simulink model "Model_Evaluation"  (R2021b)
settings: Solver=VariableStepAuto  StartTime=0.0  StopTime=10.0  RelTol=1e-3
settings Model: Creator=travispaul  LastModifiedBy=travispaul

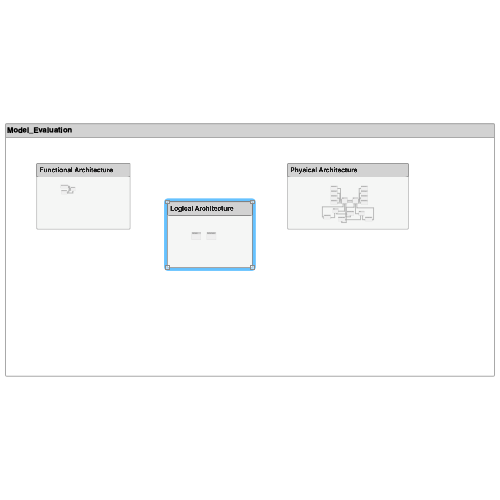
[thumbnail: Simulink's stored preview of the top-level diagram]
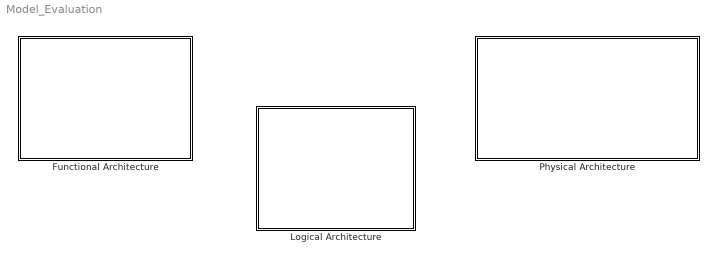
== system Model_Evaluation ==
  Functional Architecture : Subsystem
      settings: PortSchema="{\"entries\":[{\"content\":{\"headerSize\":26,\"margin\":15,\"minimumSpacing\":25,\"sides\":[{\"content\":{\"connectorIds\":[]},\"type\":\"ConnectorPlacement.EquallySpacedRectSide\",\"uuid\":\"40f43dd4-d871-4ec4-b3fe-13d7cd611bac\"},{\"content\":{\"connectorIds\":[],\"side\":\"RIGHT\"},\"type\":\"ConnectorPlacement.EquallySpacedRectSide\",\"uuid\":\"f931b331-3cfe-490c-8e42-e662817cbd7c\"},{\"content\":{\"connectorIds\":[],\"side\":\"TOP\"},\"type\":\"ConnectorPlacement.EquallySpacedRectSide\",\"uuid\":\"175320fb-a01d-4f5a-a2c2-6f21c6d50255\"}]},\"type\":\"ConnectorPlacement.EquallySpacedConnector\",\"uuid\":\"e178f2bb-de74-4782-8dfe-2993ee10560e\"}],\"packageUris\":[\"http://schema.mathworks.com/mf0/Connector/R2020b\"],\"version\":\"1.0\"}"
  Logical Architecture : Subsystem
      settings: PortSchema="{\"entries\":[{\"content\":{\"headerSize\":26,\"margin\":15,\"minimumSpacing\":25,\"sides\":[{\"content\":{\"connectorIds\":[]},\"type\":\"ConnectorPlacement.EquallySpacedRectSide\",\"uuid\":\"40f43dd4-d871-4ec4-b3fe-13d7cd611bac\"},{\"content\":{\"connectorIds\":[],\"side\":\"RIGHT\"},\"type\":\"ConnectorPlacement.EquallySpacedRectSide\",\"uuid\":\"f931b331-3cfe-490c-8e42-e662817cbd7c\"},{\"content\":{\"connectorIds\":[],\"side\":\"TOP\"},\"type\":\"ConnectorPlacement.EquallySpacedRectSide\",\"uuid\":\"175320fb-a01d-4f5a-a2c2-6f21c6d50255\"}]},\"type\":\"ConnectorPlacement.EquallySpacedConnector\",\"uuid\":\"e178f2bb-de74-4782-8dfe-2993ee10560e\"}],\"packageUris\":[\"http://schema.mathworks.com/mf0/Connector/R2020b\"],\"version\":\"1.0\"}"
  Physical Architecture : Subsystem
      settings: PortSchema="{\"entries\":[{\"content\":{\"headerSize\":26,\"margin\":15,\"minimumSpacing\":25,\"sides\":[{\"content\":{\"connectorIds\":[]},\"type\":\"ConnectorPlacement.EquallySpacedRectSide\",\"uuid\":\"40f43dd4-d871-4ec4-b3fe-13d7cd611bac\"},{\"content\":{\"connectorIds\":[],\"side\":\"RIGHT\"},\"type\":\"ConnectorPlacement.EquallySpacedRectSide\",\"uuid\":\"f931b331-3cfe-490c-8e42-e662817cbd7c\"},{\"content\":{\"connectorIds\":[],\"side\":\"TOP\"},\"type\":\"ConnectorPlacement.EquallySpacedRectSide\",\"uuid\":\"175320fb-a01d-4f5a-a2c2-6f21c6d50255\"}]},\"type\":\"ConnectorPlacement.EquallySpacedConnector\",\"uuid\":\"e178f2bb-de74-4782-8dfe-2993ee10560e\"}],\"packageUris\":[\"http://schema.mathworks.com/mf0/Connector/R2020b\"],\"version\":\"1.0\"}"

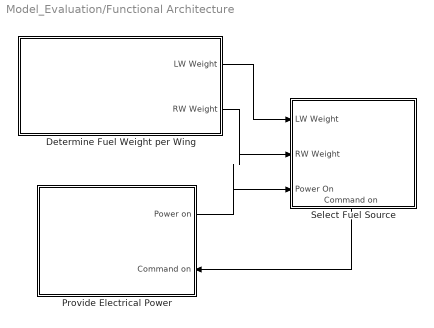
== system Model_Evaluation/Functional Architecture ==
  " Determine Fuel Weight per Wing" : Subsystem
      settings: PortSchema="{\"entries\":[{\"content\":{\"headerSize\":26,\"margin\":15,\"minimumSpacing\":25,\"sides\":[{\"content\":{\"connectorIds\":[]},\"type\":\"ConnectorPlacement.EquallySpacedRectSide\",\"uuid\":\"40f43dd4-d871-4ec4-b3fe-13d7cd611bac\"},{\"content\":{\"connectorIds\":[\"Out1\",\"Out2\"],\"side\":\"RIGHT\"},\"type\":\"ConnectorPlacement.EquallySpacedRectSide\",\"uuid\":\"f931b331-3cfe-490c-8e42-e662817cbd7c\"},{\"content\":{\"connectorIds\":[],\"side\":\"TOP\"},\"type\":\"ConnectorPlacement.EquallySpacedRectSide\",\"uuid\":\"175320fb-a01d-4f5a-a2c2-6f21c6d50255\"}]},\"type\":\"ConnectorPlacement.EquallySpacedConnector\",\"uuid\":\"e178f2bb-de74-4782-8dfe-2993ee10560e\"}],\"packageUris\":[\"http://schema.mathworks.com/mf0/Connector/R2020b\"],\"version\":\"1.0\"}"
  Provide Electrical Power : Subsystem
      settings: PortSchema="{\"entries\":[{\"content\":{\"headerSize\":26,\"margin\":15,\"minimumSpacing\":25,\"sides\":[{\"content\":{\"connectorIds\":[]},\"type\":\"ConnectorPlacement.EquallySpacedRectSide\",\"uuid\":\"40f43dd4-d871-4ec4-b3fe-13d7cd611bac\"},{\"content\":{\"connectorIds\":[\"Out1\",\"In1\"],\"side\":\"RIGHT\"},\"type\":\"ConnectorPlacement.EquallySpacedRectSide\",\"uuid\":\"f931b331-3cfe-490c-8e42-e662817cbd7c\"},{\"content\":{\"connectorIds\":[],\"side\":\"TOP\"},\"type\":\"ConnectorPlacement.EquallySpacedRectSide\",\"uuid\":\"175320fb-a01d-4f5a-a2c2-6f21c6d50255\"}]},\"type\":\"ConnectorPlacement.EquallySpacedConnector\",\"uuid\":\"e178f2bb-de74-4782-8dfe-2993ee10560e\"}],\"packageUris\":[\"http://schema.mathworks.com/mf0/Connector/R2020b\"],\"version\":\"1.0\"}"
  Select Fuel Source : Subsystem
      settings: PortSchema="{\"entries\":[{\"content\":{\"headerSize\":26,\"margin\":15,\"minimumSpacing\":25,\"sides\":[{\"content\":{\"connectorIds\":[\"In1\",\"In2\",\"In3\"]},\"type\":\"ConnectorPlacement.EquallySpacedRectSide\",\"uuid\":\"40f43dd4-d871-4ec4-b3fe-13d7cd611bac\"},{\"content\":{\"connectorIds\":[],\"side\":\"RIGHT\"},\"type\":\"ConnectorPlacement.EquallySpacedRectSide\",\"uuid\":\"f931b331-3cfe-490c-8e42-e662817cbd7c\"},{\"content\":{\"connectorIds\":[],\"side\":\"TOP\"},\"type\":\"ConnectorPlacement.EquallySpacedRectSide\",\"uuid\":\"175320fb-a01d-4f5a-a2c2-6f21c6d50255\"},{\"content\":{\"connectorIds\":[\"Out1\"],\"side\":\"BOTTOM\"},\"type\":\"ConnectorPlacement.EquallySpacedRectSide\",\"uuid\":\"3de24a88-b66c-416d-81ff-fa8204919022\"}]},\"type\":\"ConnectorPlacement.EquallySpacedConnector\",\"uuid\":\"e178f2bb-de74-4782-8dfe-2993ee10560e\"}],\"packageUris\":[\"http://schema.mathworks.com/mf0/Connector/R2020b\"],\"version\":\"1.0\"}"
  wires:
  " Determine Fuel Weight per Wing"/2(RW Weight) -> Select Fuel Source/2(RW Weight)
  Provide Electrical Power/1(Power on) -> Select Fuel Source/3(Power On)
  " Determine Fuel Weight per Wing"/1(LW Weight) -> Select Fuel Source/1(LW Weight)
  Select Fuel Source/1(Command on) -> Provide Electrical Power/1(Command on)

== system Model_Evaluation/Logical Architecture ==
  Electrical System : Subsystem
      settings: PortSchema="{\"entries\":[{\"content\":{\"headerSize\":26,\"margin\":15,\"minimumSpacing\":25,\"sides\":[{\"content\":{\"connectorIds\":[]},\"type\":\"ConnectorPlacement.EquallySpacedRectSide\",\"uuid\":\"40f43dd4-d871-4ec4-b3fe-13d7cd611bac\"},{\"content\":{\"connectorIds\":[],\"side\":\"RIGHT\"},\"type\":\"ConnectorPlacement.EquallySpacedRectSide\",\"uuid\":\"f931b331-3cfe-490c-8e42-e662817cbd7c\"},{\"content\":{\"connectorIds\":[],\"side\":\"TOP\"},\"type\":\"ConnectorPlacement.EquallySpacedRectSide\",\"uuid\":\"175320fb-a01d-4f5a-a2c2-6f21c6d50255\"}]},\"type\":\"ConnectorPlacement.EquallySpacedConnector\",\"uuid\":\"e178f2bb-de74-4782-8dfe-2993ee10560e\"}],\"packageUris\":[\"http://schema.mathworks.com/mf0/Connector/R2020b\"],\"version\":\"1.0\"}"
  Fuel System : Subsystem
      settings: PortSchema="{\"entries\":[{\"content\":{\"headerSize\":26,\"margin\":15,\"minimumSpacing\":25,\"sides\":[{\"content\":{\"connectorIds\":[]},\"type\":\"ConnectorPlacement.EquallySpacedRectSide\",\"uuid\":\"40f43dd4-d871-4ec4-b3fe-13d7cd611bac\"},{\"content\":{\"connectorIds\":[],\"side\":\"RIGHT\"},\"type\":\"ConnectorPlacement.EquallySpacedRectSide\",\"uuid\":\"f931b331-3cfe-490c-8e42-e662817cbd7c\"},{\"content\":{\"connectorIds\":[],\"side\":\"TOP\"},\"type\":\"ConnectorPlacement.EquallySpacedRectSide\",\"uuid\":\"175320fb-a01d-4f5a-a2c2-6f21c6d50255\"}]},\"type\":\"ConnectorPlacement.EquallySpacedConnector\",\"uuid\":\"e178f2bb-de74-4782-8dfe-2993ee10560e\"}],\"packageUris\":[\"http://schema.mathworks.com/mf0/Connector/R2020b\"],\"version\":\"1.0\"}"

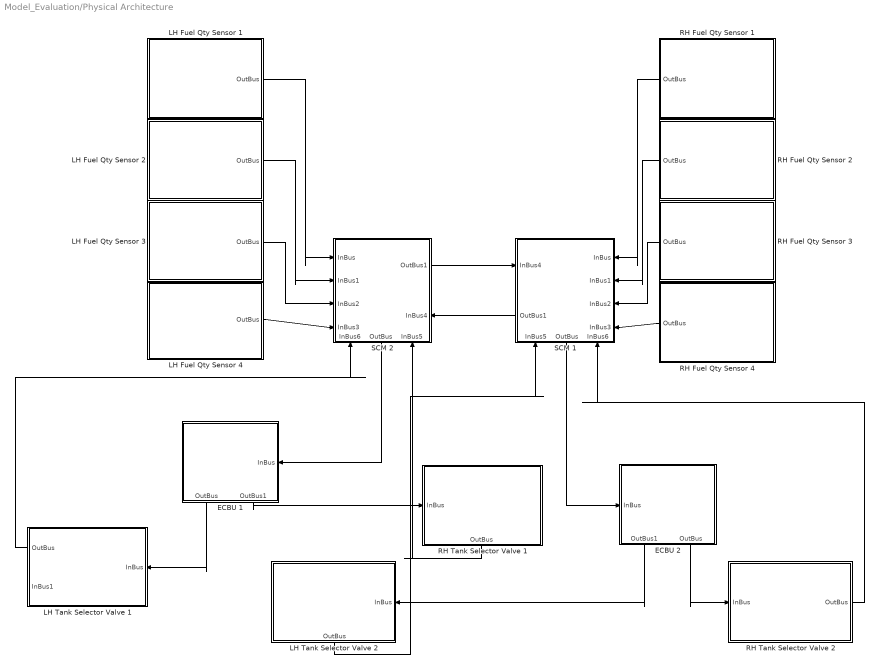
== system Model_Evaluation/Physical Architecture ==
  ECBU 1 : Subsystem
      settings: PortSchema="{\"entries\":[{\"content\":{\"headerSize\":26,\"margin\":15,\"minimumSpacing\":25,\"sides\":[{\"content\":{\"connectorIds\":[]},\"type\":\"ConnectorPlacement.EquallySpacedRectSide\",\"uuid\":\"40f43dd4-d871-4ec4-b3fe-13d7cd611bac\"},{\"content\":{\"connectorIds\":[\"In1\"],\"side\":\"RIGHT\"},\"type\":\"ConnectorPlacement.EquallySpacedRectSide\",\"uuid\":\"f931b331-3cfe-490c-8e42-e662817cbd7c\"},{\"content\":{\"connectorIds\":[],\"side\":\"TOP\"},\"type\":\"ConnectorPlacement.EquallySpacedRectSide\",\"uuid\":\"175320fb-a01d-4f5a-a2c2-6f21c6d50255\"},{\"content\":{\"connectorIds\":[\"Out1\",\"Out2\"],\"side\":\"BOTTOM\"},\"type\":\"ConnectorPlacement.EquallySpacedRectSide\",\"uuid\":\"fddd49d8-f2b5-4282-8669-7c84809d93ad\"}]},\"type\":\"ConnectorPlacement.EquallySpacedConnector\",\"uuid\":\"e178f2bb-de74-4782-8dfe-2993ee10560e\"}],\"packageUris\":[\"http://schema.mathworks.com/mf0/Connector/R2020b\"],\"version\":\"1.0\"}"
  ECBU 2 : Subsystem
      settings: PortSchema="{\"entries\":[{\"content\":{\"headerSize\":26,\"margin\":15,\"minimumSpacing\":25,\"sides\":[{\"content\":{\"connectorIds\":[\"In1\"]},\"type\":\"ConnectorPlacement.EquallySpacedRectSide\",\"uuid\":\"40f43dd4-d871-4ec4-b3fe-13d7cd611bac\"},{\"content\":{\"connectorIds\":[],\"side\":\"RIGHT\"},\"type\":\"ConnectorPlacement.EquallySpacedRectSide\",\"uuid\":\"f931b331-3cfe-490c-8e42-e662817cbd7c\"},{\"content\":{\"connectorIds\":[],\"side\":\"TOP\"},\"type\":\"ConnectorPlacement.EquallySpacedRectSide\",\"uuid\":\"175320fb-a01d-4f5a-a2c2-6f21c6d50255\"},{\"content\":{\"connectorIds\":[\"Out1\",\"Out2\"],\"side\":\"BOTTOM\"},\"type\":\"ConnectorPlacement.EquallySpacedRectSide\",\"uuid\":\"1da1c11c-311b-49b1-a7e1-1e0e53e00fa4\"}]},\"type\":\"ConnectorPlacement.EquallySpacedConnector\",\"uuid\":\"e178f2bb-de74-4782-8dfe-2993ee10560e\"}],\"packageUris\":[\"http://schema.mathworks.com/mf0/Connector/R2020b\"],\"version\":\"1.0\"}"
  LH Fuel Qty Sensor 1 : Subsystem
      settings: PortSchema="{\"entries\":[{\"content\":{\"headerSize\":26,\"margin\":15,\"minimumSpacing\":25,\"sides\":[{\"content\":{\"connectorIds\":[]},\"type\":\"ConnectorPlacement.EquallySpacedRectSide\",\"uuid\":\"40f43dd4-d871-4ec4-b3fe-13d7cd611bac\"},{\"content\":{\"connectorIds\":[\"Out1\"],\"side\":\"RIGHT\"},\"type\":\"ConnectorPlacement.EquallySpacedRectSide\",\"uuid\":\"f931b331-3cfe-490c-8e42-e662817cbd7c\"},{\"content\":{\"connectorIds\":[],\"side\":\"TOP\"},\"type\":\"ConnectorPlacement.EquallySpacedRectSide\",\"uuid\":\"175320fb-a01d-4f5a-a2c2-6f21c6d50255\"}]},\"type\":\"ConnectorPlacement.EquallySpacedConnector\",\"uuid\":\"e178f2bb-de74-4782-8dfe-2993ee10560e\"}],\"packageUris\":[\"http://schema.mathworks.com/mf0/Connector/R2020b\"],\"version\":\"1.0\"}"
  LH Fuel Qty Sensor 2 : Subsystem
      settings: PortSchema="{\"entries\":[{\"content\":{\"headerSize\":26,\"margin\":15,\"minimumSpacing\":25,\"sides\":[{\"content\":{\"connectorIds\":[]},\"type\":\"ConnectorPlacement.EquallySpacedRectSide\",\"uuid\":\"40f43dd4-d871-4ec4-b3fe-13d7cd611bac\"},{\"content\":{\"connectorIds\":[\"Out1\"],\"side\":\"RIGHT\"},\"type\":\"ConnectorPlacement.EquallySpacedRectSide\",\"uuid\":\"f931b331-3cfe-490c-8e42-e662817cbd7c\"},{\"content\":{\"connectorIds\":[],\"side\":\"TOP\"},\"type\":\"ConnectorPlacement.EquallySpacedRectSide\",\"uuid\":\"175320fb-a01d-4f5a-a2c2-6f21c6d50255\"}]},\"type\":\"ConnectorPlacement.EquallySpacedConnector\",\"uuid\":\"e178f2bb-de74-4782-8dfe-2993ee10560e\"}],\"packageUris\":[\"http://schema.mathworks.com/mf0/Connector/R2020b\"],\"version\":\"1.0\"}"
  LH Fuel Qty Sensor 3 : Subsystem
      settings: PortSchema="{\"entries\":[{\"content\":{\"headerSize\":26,\"margin\":15,\"minimumSpacing\":25,\"sides\":[{\"content\":{\"connectorIds\":[]},\"type\":\"ConnectorPlacement.EquallySpacedRectSide\",\"uuid\":\"40f43dd4-d871-4ec4-b3fe-13d7cd611bac\"},{\"content\":{\"connectorIds\":[\"Out1\"],\"side\":\"RIGHT\"},\"type\":\"ConnectorPlacement.EquallySpacedRectSide\",\"uuid\":\"f931b331-3cfe-490c-8e42-e662817cbd7c\"},{\"content\":{\"connectorIds\":[],\"side\":\"TOP\"},\"type\":\"ConnectorPlacement.EquallySpacedRectSide\",\"uuid\":\"175320fb-a01d-4f5a-a2c2-6f21c6d50255\"}]},\"type\":\"ConnectorPlacement.EquallySpacedConnector\",\"uuid\":\"e178f2bb-de74-4782-8dfe-2993ee10560e\"}],\"packageUris\":[\"http://schema.mathworks.com/mf0/Connector/R2020b\"],\"version\":\"1.0\"}"
  LH Fuel Qty Sensor 4 : Subsystem
      settings: PortSchema="{\"entries\":[{\"content\":{\"headerSize\":26,\"margin\":15,\"minimumSpacing\":25,\"sides\":[{\"content\":{\"connectorIds\":[]},\"type\":\"ConnectorPlacement.EquallySpacedRectSide\",\"uuid\":\"40f43dd4-d871-4ec4-b3fe-13d7cd611bac\"},{\"content\":{\"connectorIds\":[\"Out1\"],\"side\":\"RIGHT\"},\"type\":\"ConnectorPlacement.EquallySpacedRectSide\",\"uuid\":\"f931b331-3cfe-490c-8e42-e662817cbd7c\"},{\"content\":{\"connectorIds\":[],\"side\":\"TOP\"},\"type\":\"ConnectorPlacement.EquallySpacedRectSide\",\"uuid\":\"175320fb-a01d-4f5a-a2c2-6f21c6d50255\"}]},\"type\":\"ConnectorPlacement.EquallySpacedConnector\",\"uuid\":\"e178f2bb-de74-4782-8dfe-2993ee10560e\"}],\"packageUris\":[\"http://schema.mathworks.com/mf0/Connector/R2020b\"],\"version\":\"1.0\"}"
  LH Tank Selector Valve 1 : Subsystem
      settings: PortSchema="{\"entries\":[{\"content\":{\"headerSize\":26,\"margin\":15,\"minimumSpacing\":25,\"sides\":[{\"content\":{\"connectorIds\":[\"Out1\",\"In1\"]},\"type\":\"ConnectorPlacement.EquallySpacedRectSide\",\"uuid\":\"40f43dd4-d871-4ec4-b3fe-13d7cd611bac\"},{\"content\":{\"connectorIds\":[\"In2\"],\"side\":\"RIGHT\"},\"type\":\"ConnectorPlacement.EquallySpacedRectSide\",\"uuid\":\"f931b331-3cfe-490c-8e42-e662817cbd7c\"},{\"content\":{\"connectorIds\":[],\"side\":\"TOP\"},\"type\":\"ConnectorPlacement.EquallySpacedRectSide\",\"uuid\":\"175320fb-a01d-4f5a-a2c2-6f21c6d50255\"}]},\"type\":\"ConnectorPlacement.EquallySpacedConnector\",\"uuid\":\"e178f2bb-de74-4782-8dfe-2993ee10560e\"}],\"packageUris\":[\"http://schema.mathworks.com/mf0/Connector/R2020b\"],\"version\":\"1.0\"}"
  LH Tank Selector Valve 2 : Subsystem
      settings: PortSchema="{\"entries\":[{\"content\":{\"headerSize\":26,\"margin\":15,\"minimumSpacing\":25,\"sides\":[{\"content\":{\"connectorIds\":[]},\"type\":\"ConnectorPlacement.EquallySpacedRectSide\",\"uuid\":\"40f43dd4-d871-4ec4-b3fe-13d7cd611bac\"},{\"content\":{\"connectorIds\":[\"In1\"],\"side\":\"RIGHT\"},\"type\":\"ConnectorPlacement.EquallySpacedRectSide\",\"uuid\":\"f931b331-3cfe-490c-8e42-e662817cbd7c\"},{\"content\":{\"connectorIds\":[],\"side\":\"TOP\"},\"type\":\"ConnectorPlacement.EquallySpacedRectSide\",\"uuid\":\"175320fb-a01d-4f5a-a2c2-6f21c6d50255\"},{\"content\":{\"connectorIds\":[\"Out1\"],\"side\":\"BOTTOM\"},\"type\":\"ConnectorPlacement.EquallySpacedRectSide\",\"uuid\":\"36eb773b-40b4-4869-82f1-a932584a6324\"}]},\"type\":\"ConnectorPlacement.EquallySpacedConnector\",\"uuid\":\"e178f2bb-de74-4782-8dfe-2993ee10560e\"}],\"packageUris\":[\"http://schema.mathworks.com/mf0/Connector/R2020b\"],\"version\":\"1.0\"}"
  RH Fuel Qty Sensor 1 : Subsystem
      settings: PortSchema="{\"entries\":[{\"content\":{\"headerSize\":26,\"margin\":15,\"minimumSpacing\":25,\"sides\":[{\"content\":{\"connectorIds\":[\"Out1\"]},\"type\":\"ConnectorPlacement.EquallySpacedRectSide\",\"uuid\":\"40f43dd4-d871-4ec4-b3fe-13d7cd611bac\"},{\"content\":{\"connectorIds\":[],\"side\":\"RIGHT\"},\"type\":\"ConnectorPlacement.EquallySpacedRectSide\",\"uuid\":\"f931b331-3cfe-490c-8e42-e662817cbd7c\"},{\"content\":{\"connectorIds\":[],\"side\":\"TOP\"},\"type\":\"ConnectorPlacement.EquallySpacedRectSide\",\"uuid\":\"175320fb-a01d-4f5a-a2c2-6f21c6d50255\"},{\"content\":{\"connectorIds\":[],\"side\":\"BOTTOM\"},\"type\":\"ConnectorPlacement.EquallySpacedRectSide\",\"uuid\":\"fd82acf4-c674-4780-980d-bd8d3c341496\"}]},\"type\":\"ConnectorPlacement.EquallySpacedConnector\",\"uuid\":\"e178f2bb-de74-4782-8dfe-2993ee10560e\"}],\"packageUris\":[\"http://schema.mathworks.com/mf0/Connector/R2020b\"],\"version\":\"1.0\"}"
  RH Fuel Qty Sensor 2 : Subsystem
      settings: PortSchema="{\"entries\":[{\"content\":{\"headerSize\":26,\"margin\":15,\"minimumSpacing\":25,\"sides\":[{\"content\":{\"connectorIds\":[\"Out1\"]},\"type\":\"ConnectorPlacement.EquallySpacedRectSide\",\"uuid\":\"40f43dd4-d871-4ec4-b3fe-13d7cd611bac\"},{\"content\":{\"connectorIds\":[],\"side\":\"RIGHT\"},\"type\":\"ConnectorPlacement.EquallySpacedRectSide\",\"uuid\":\"f931b331-3cfe-490c-8e42-e662817cbd7c\"},{\"content\":{\"connectorIds\":[],\"side\":\"TOP\"},\"type\":\"ConnectorPlacement.EquallySpacedRectSide\",\"uuid\":\"175320fb-a01d-4f5a-a2c2-6f21c6d50255\"},{\"content\":{\"connectorIds\":[],\"side\":\"BOTTOM\"},\"type\":\"ConnectorPlacement.EquallySpacedRectSide\",\"uuid\":\"db131b08-d750-4d9e-b7a5-2b13541e51b6\"}]},\"type\":\"ConnectorPlacement.EquallySpacedConnector\",\"uuid\":\"e178f2bb-de74-4782-8dfe-2993ee10560e\"}],\"packageUris\":[\"http://schema.mathworks.com/mf0/Connector/R2020b\"],\"version\":\"1.0\"}"
  RH Fuel Qty Sensor 3 : Subsystem
      settings: PortSchema="{\"entries\":[{\"content\":{\"headerSize\":26,\"margin\":15,\"minimumSpacing\":25,\"sides\":[{\"content\":{\"connectorIds\":[\"Out1\"]},\"type\":\"ConnectorPlacement.EquallySpacedRectSide\",\"uuid\":\"40f43dd4-d871-4ec4-b3fe-13d7cd611bac\"},{\"content\":{\"connectorIds\":[],\"side\":\"RIGHT\"},\"type\":\"ConnectorPlacement.EquallySpacedRectSide\",\"uuid\":\"f931b331-3cfe-490c-8e42-e662817cbd7c\"},{\"content\":{\"connectorIds\":[],\"side\":\"TOP\"},\"type\":\"ConnectorPlacement.EquallySpacedRectSide\",\"uuid\":\"175320fb-a01d-4f5a-a2c2-6f21c6d50255\"},{\"content\":{\"connectorIds\":[],\"side\":\"BOTTOM\"},\"type\":\"ConnectorPlacement.EquallySpacedRectSide\",\"uuid\":\"88848ca8-7028-48d0-962f-017e01948154\"}]},\"type\":\"ConnectorPlacement.EquallySpacedConnector\",\"uuid\":\"e178f2bb-de74-4782-8dfe-2993ee10560e\"}],\"packageUris\":[\"http://schema.mathworks.com/mf0/Connector/R2020b\"],\"version\":\"1.0\"}"
  RH Fuel Qty Sensor 4 : Subsystem
      settings: PortSchema="{\"entries\":[{\"content\":{\"headerSize\":26,\"margin\":15,\"minimumSpacing\":25,\"sides\":[{\"content\":{\"connectorIds\":[\"Out1\"]},\"type\":\"ConnectorPlacement.EquallySpacedRectSide\",\"uuid\":\"40f43dd4-d871-4ec4-b3fe-13d7cd611bac\"},{\"content\":{\"connectorIds\":[],\"side\":\"RIGHT\"},\"type\":\"ConnectorPlacement.EquallySpacedRectSide\",\"uuid\":\"f931b331-3cfe-490c-8e42-e662817cbd7c\"},{\"content\":{\"connectorIds\":[],\"side\":\"TOP\"},\"type\":\"ConnectorPlacement.EquallySpacedRectSide\",\"uuid\":\"175320fb-a01d-4f5a-a2c2-6f21c6d50255\"},{\"content\":{\"connectorIds\":[],\"side\":\"BOTTOM\"},\"type\":\"ConnectorPlacement.EquallySpacedRectSide\",\"uuid\":\"7f3ee34d-6c00-486b-97ca-d8decc164e9c\"}]},\"type\":\"ConnectorPlacement.EquallySpacedConnector\",\"uuid\":\"e178f2bb-de74-4782-8dfe-2993ee10560e\"}],\"packageUris\":[\"http://schema.mathworks.com/mf0/Connector/R2020b\"],\"version\":\"1.0\"}"
  RH Tank Selector Valve 1 : Subsystem
      settings: PortSchema="{\"entries\":[{\"content\":{\"headerSize\":26,\"margin\":15,\"minimumSpacing\":25,\"sides\":[{\"content\":{\"connectorIds\":[\"In1\"]},\"type\":\"ConnectorPlacement.EquallySpacedRectSide\",\"uuid\":\"40f43dd4-d871-4ec4-b3fe-13d7cd611bac\"},{\"content\":{\"connectorIds\":[],\"side\":\"RIGHT\"},\"type\":\"ConnectorPlacement.EquallySpacedRectSide\",\"uuid\":\"f931b331-3cfe-490c-8e42-e662817cbd7c\"},{\"content\":{\"connectorIds\":[],\"side\":\"TOP\"},\"type\":\"ConnectorPlacement.EquallySpacedRectSide\",\"uuid\":\"175320fb-a01d-4f5a-a2c2-6f21c6d50255\"},{\"content\":{\"connectorIds\":[\"Out1\"],\"side\":\"BOTTOM\"},\"type\":\"ConnectorPlacement.EquallySpacedRectSide\",\"uuid\":\"5e16c353-8a5f-433c-85d9-03a6f371bd75\"}]},\"type\":\"ConnectorPlacement.EquallySpacedConnector\",\"uuid\":\"e178f2bb-de74-4782-8dfe-2993ee10560e\"}],\"packageUris\":[\"http://schema.mathworks.com/mf0/Connector/R2020b\"],\"version\":\"1.0\"}"
  RH Tank Selector Valve 2 : Subsystem
      settings: PortSchema="{\"entries\":[{\"content\":{\"headerSize\":26,\"margin\":15,\"minimumSpacing\":25,\"sides\":[{\"content\":{\"connectorIds\":[\"In1\"]},\"type\":\"ConnectorPlacement.EquallySpacedRectSide\",\"uuid\":\"40f43dd4-d871-4ec4-b3fe-13d7cd611bac\"},{\"content\":{\"connectorIds\":[\"Out1\"],\"side\":\"RIGHT\"},\"type\":\"ConnectorPlacement.EquallySpacedRectSide\",\"uuid\":\"f931b331-3cfe-490c-8e42-e662817cbd7c\"},{\"content\":{\"connectorIds\":[],\"side\":\"TOP\"},\"type\":\"ConnectorPlacement.EquallySpacedRectSide\",\"uuid\":\"175320fb-a01d-4f5a-a2c2-6f21c6d50255\"}]},\"type\":\"ConnectorPlacement.EquallySpacedConnector\",\"uuid\":\"e178f2bb-de74-4782-8dfe-2993ee10560e\"}],\"packageUris\":[\"http://schema.mathworks.com/mf0/Connector/R2020b\"],\"version\":\"1.0\"}"
  SCM 1 : Subsystem
      settings: PortSchema="{\"entries\":[{\"content\":{\"headerSize\":26,\"margin\":15,\"minimumSpacing\":25,\"sides\":[{\"content\":{\"connectorIds\":[\"In3\",\"Out1\"]},\"type\":\"ConnectorPlacement.EquallySpacedRectSide\",\"uuid\":\"40f43dd4-d871-4ec4-b3fe-13d7cd611bac\"},{\"content\":{\"connectorIds\":[\"In4\",\"In5\",\"In6\",\"In7\"],\"side\":\"RIGHT\"},\"type\":\"ConnectorPlacement.EquallySpacedRectSide\",\"uuid\":\"f931b331-3cfe-490c-8e42-e662817cbd7c\"},{\"content\":{\"connectorIds\":[],\"side\":\"TOP\"},\"type\":\"ConnectorPlacement.EquallySpacedRectSide\",\"uuid\":\"175320fb-a01d-4f5a-a2c2-6f21c6d50255\"},{\"content\":{\"connectorIds\":[\"In1\",\"Out2\",\"In2\"],\"side\":\"BOTTOM\"},\"type\":\"ConnectorPlacement.EquallySpacedRectSide\",\"uuid\":\"d21d2942-17a9-430e-ace1-94ca6a721bab\"}]},\"type\":\"ConnectorPlacement.EquallySpacedConnector\",\"uuid\":\"e178f2bb-de74-4782-8dfe-2993ee10560e\"}],\"packageUris\":[\"http://schema.mathworks.com/mf0/Connector/R2020b\"],\"version\":\"1.0\"}"
  SCM 2 : Subsystem
      settings: PortSchema="{\"entries\":[{\"content\":{\"headerSize\":26,\"margin\":15,\"minimumSpacing\":25,\"sides\":[{\"content\":{\"connectorIds\":[\"In4\",\"In5\",\"In6\",\"In7\"]},\"type\":\"ConnectorPlacement.EquallySpacedRectSide\",\"uuid\":\"40f43dd4-d871-4ec4-b3fe-13d7cd611bac\"},{\"content\":{\"connectorIds\":[\"Out1\",\"In3\"],\"side\":\"RIGHT\"},\"type\":\"ConnectorPlacement.EquallySpacedRectSide\",\"uuid\":\"f931b331-3cfe-490c-8e42-e662817cbd7c\"},{\"content\":{\"connectorIds\":[],\"side\":\"TOP\"},\"type\":\"ConnectorPlacement.EquallySpacedRectSide\",\"uuid\":\"175320fb-a01d-4f5a-a2c2-6f21c6d50255\"},{\"content\":{\"connectorIds\":[\"In1\",\"Out2\",\"In2\"],\"side\":\"BOTTOM\"},\"type\":\"ConnectorPlacement.EquallySpacedRectSide\",\"uuid\":\"8f956892-5c7b-4f02-b39a-e9441250dc4b\"}]},\"type\":\"ConnectorPlacement.EquallySpacedConnector\",\"uuid\":\"e178f2bb-de74-4782-8dfe-2993ee10560e\"}],\"packageUris\":[\"http://schema.mathworks.com/mf0/Connector/R2020b\"],\"version\":\"1.0\"}"
  wires:
  LH Fuel Qty Sensor 1/1(OutBus) -> SCM 2/4(InBus)
  LH Fuel Qty Sensor 2/1(OutBus) -> SCM 2/5(InBus1)
  LH Fuel Qty Sensor 3/1(OutBus) -> SCM 2/6(InBus2)
  LH Fuel Qty Sensor 4/1(OutBus) -> SCM 2/7(InBus3)
  RH Fuel Qty Sensor 1/1(OutBus) -> SCM 1/4(InBus)
  RH Fuel Qty Sensor 2/1(OutBus) -> SCM 1/5(InBus1)
  RH Fuel Qty Sensor 3/1(OutBus) -> SCM 1/6(InBus2)
  RH Fuel Qty Sensor 4/1(OutBus) -> SCM 1/7(InBus3)
  SCM 1/2(OutBus) -> ECBU 2/1(InBus)
  SCM 2/2(OutBus) -> ECBU 1/1(InBus)
  ECBU 1/1(OutBus) -> LH Tank Selector Valve 1/2(InBus)
  ECBU 1/2(OutBus1) -> RH Tank Selector Valve 1/1(InBus)
  ECBU 2/2(OutBus) -> RH Tank Selector Valve 2/1(InBus)
  ECBU 2/1(OutBus1) -> LH Tank Selector Valve 2/1(InBus)
  SCM 2/1(OutBus1) -> SCM 1/3(InBus4)
  SCM 1/1(OutBus1) -> SCM 2/3(InBus4)
  RH Tank Selector Valve 1/1(OutBus) -> SCM 2/2(InBus5)
  LH Tank Selector Valve 2/1(OutBus) -> SCM 1/1(InBus5)
  RH Tank Selector Valve 2/1(OutBus) -> SCM 1/2(InBus6)
  LH Tank Selector Valve 1/1(OutBus) -> SCM 2/1(InBus6)

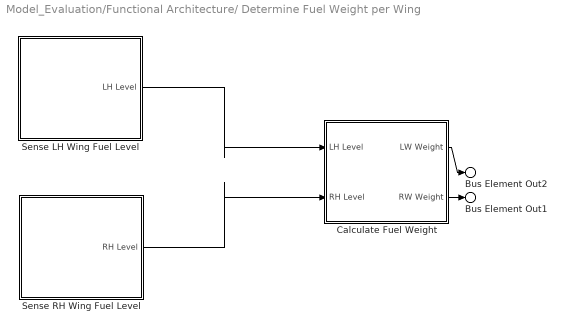
== system Model_Evaluation/Functional Architecture/ Determine Fuel Weight per Wing ==
  Calculate Fuel Weight : Subsystem
      settings: PortSchema="{\"entries\":[{\"content\":{\"headerSize\":26,\"margin\":15,\"minimumSpacing\":25,\"sides\":[{\"content\":{\"connectorIds\":[\"In1\",\"In2\"]},\"type\":\"ConnectorPlacement.EquallySpacedRectSide\",\"uuid\":\"40f43dd4-d871-4ec4-b3fe-13d7cd611bac\"},{\"content\":{\"connectorIds\":[\"Out1\",\"Out2\"],\"side\":\"RIGHT\"},\"type\":\"ConnectorPlacement.EquallySpacedRectSide\",\"uuid\":\"f931b331-3cfe-490c-8e42-e662817cbd7c\"},{\"content\":{\"connectorIds\":[],\"side\":\"TOP\"},\"type\":\"ConnectorPlacement.EquallySpacedRectSide\",\"uuid\":\"175320fb-a01d-4f5a-a2c2-6f21c6d50255\"}]},\"type\":\"ConnectorPlacement.EquallySpacedConnector\",\"uuid\":\"e178f2bb-de74-4782-8dfe-2993ee10560e\"}],\"packageUris\":[\"http://schema.mathworks.com/mf0/Connector/R2020b\"],\"version\":\"1.0\"}"
  Sense LH Wing Fuel Level : Subsystem
      settings: PortSchema="{\"entries\":[{\"content\":{\"headerSize\":26,\"margin\":15,\"minimumSpacing\":25,\"sides\":[{\"content\":{\"connectorIds\":[]},\"type\":\"ConnectorPlacement.EquallySpacedRectSide\",\"uuid\":\"40f43dd4-d871-4ec4-b3fe-13d7cd611bac\"},{\"content\":{\"connectorIds\":[\"Out1\"],\"side\":\"RIGHT\"},\"type\":\"ConnectorPlacement.EquallySpacedRectSide\",\"uuid\":\"f931b331-3cfe-490c-8e42-e662817cbd7c\"},{\"content\":{\"connectorIds\":[],\"side\":\"TOP\"},\"type\":\"ConnectorPlacement.EquallySpacedRectSide\",\"uuid\":\"175320fb-a01d-4f5a-a2c2-6f21c6d50255\"}]},\"type\":\"ConnectorPlacement.EquallySpacedConnector\",\"uuid\":\"e178f2bb-de74-4782-8dfe-2993ee10560e\"}],\"packageUris\":[\"http://schema.mathworks.com/mf0/Connector/R2020b\"],\"version\":\"1.0\"}"
  Sense RH Wing Fuel Level : Subsystem
      settings: PortSchema="{\"entries\":[{\"content\":{\"headerSize\":26,\"margin\":15,\"minimumSpacing\":25,\"sides\":[{\"content\":{\"connectorIds\":[]},\"type\":\"ConnectorPlacement.EquallySpacedRectSide\",\"uuid\":\"40f43dd4-d871-4ec4-b3fe-13d7cd611bac\"},{\"content\":{\"connectorIds\":[\"Out1\"],\"side\":\"RIGHT\"},\"type\":\"ConnectorPlacement.EquallySpacedRectSide\",\"uuid\":\"f931b331-3cfe-490c-8e42-e662817cbd7c\"},{\"content\":{\"connectorIds\":[],\"side\":\"TOP\"},\"type\":\"ConnectorPlacement.EquallySpacedRectSide\",\"uuid\":\"175320fb-a01d-4f5a-a2c2-6f21c6d50255\"}]},\"type\":\"ConnectorPlacement.EquallySpacedConnector\",\"uuid\":\"e178f2bb-de74-4782-8dfe-2993ee10560e\"}],\"packageUris\":[\"http://schema.mathworks.com/mf0/Connector/R2020b\"],\"version\":\"1.0\"}"
  Bus Element Out2 : Outport  PortName=LW Weight
  Bus Element Out1 : Outport  Port=2  PortName=RW Weight
  wires:
  Sense RH Wing Fuel Level/1(RH Level) -> Calculate Fuel Weight/2(RH Level)
  Sense LH Wing Fuel Level/1(LH Level) -> Calculate Fuel Weight/1(LH Level)
  Calculate Fuel Weight/1(LW Weight) -> Bus Element Out2/1
  Calculate Fuel Weight/2(RW Weight) -> Bus Element Out1/1

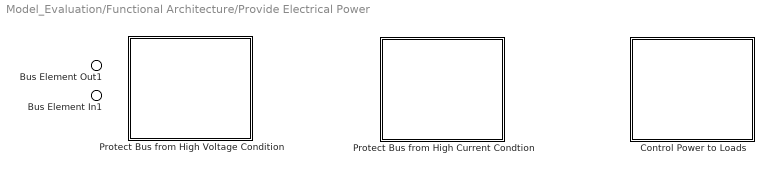
== system Model_Evaluation/Functional Architecture/Provide Electrical Power ==
  Bus Element In1 : Inport  PortName=Command on
  Control Power to Loads : Subsystem
      settings: PortSchema="{\"entries\":[{\"content\":{\"headerSize\":26,\"margin\":15,\"minimumSpacing\":25,\"sides\":[{\"content\":{\"connectorIds\":[]},\"type\":\"ConnectorPlacement.EquallySpacedRectSide\",\"uuid\":\"40f43dd4-d871-4ec4-b3fe-13d7cd611bac\"},{\"content\":{\"connectorIds\":[],\"side\":\"RIGHT\"},\"type\":\"ConnectorPlacement.EquallySpacedRectSide\",\"uuid\":\"f931b331-3cfe-490c-8e42-e662817cbd7c\"},{\"content\":{\"connectorIds\":[],\"side\":\"TOP\"},\"type\":\"ConnectorPlacement.EquallySpacedRectSide\",\"uuid\":\"175320fb-a01d-4f5a-a2c2-6f21c6d50255\"}]},\"type\":\"ConnectorPlacement.EquallySpacedConnector\",\"uuid\":\"e178f2bb-de74-4782-8dfe-2993ee10560e\"}],\"packageUris\":[\"http://schema.mathworks.com/mf0/Connector/R2020b\"],\"version\":\"1.0\"}"
  Protect Bus from High Current Condtion : Subsystem
      settings: PortSchema="{\"entries\":[{\"content\":{\"headerSize\":26,\"margin\":15,\"minimumSpacing\":25,\"sides\":[{\"content\":{\"connectorIds\":[]},\"type\":\"ConnectorPlacement.EquallySpacedRectSide\",\"uuid\":\"40f43dd4-d871-4ec4-b3fe-13d7cd611bac\"},{\"content\":{\"connectorIds\":[],\"side\":\"RIGHT\"},\"type\":\"ConnectorPlacement.EquallySpacedRectSide\",\"uuid\":\"f931b331-3cfe-490c-8e42-e662817cbd7c\"},{\"content\":{\"connectorIds\":[],\"side\":\"TOP\"},\"type\":\"ConnectorPlacement.EquallySpacedRectSide\",\"uuid\":\"175320fb-a01d-4f5a-a2c2-6f21c6d50255\"}]},\"type\":\"ConnectorPlacement.EquallySpacedConnector\",\"uuid\":\"e178f2bb-de74-4782-8dfe-2993ee10560e\"}],\"packageUris\":[\"http://schema.mathworks.com/mf0/Connector/R2020b\"],\"version\":\"1.0\"}"
  Protect Bus from High Voltage Condition : Subsystem
      settings: PortSchema="{\"entries\":[{\"content\":{\"headerSize\":26,\"margin\":15,\"minimumSpacing\":25,\"sides\":[{\"content\":{\"connectorIds\":[]},\"type\":\"ConnectorPlacement.EquallySpacedRectSide\",\"uuid\":\"40f43dd4-d871-4ec4-b3fe-13d7cd611bac\"},{\"content\":{\"connectorIds\":[],\"side\":\"RIGHT\"},\"type\":\"ConnectorPlacement.EquallySpacedRectSide\",\"uuid\":\"f931b331-3cfe-490c-8e42-e662817cbd7c\"},{\"content\":{\"connectorIds\":[],\"side\":\"TOP\"},\"type\":\"ConnectorPlacement.EquallySpacedRectSide\",\"uuid\":\"175320fb-a01d-4f5a-a2c2-6f21c6d50255\"}]},\"type\":\"ConnectorPlacement.EquallySpacedConnector\",\"uuid\":\"e178f2bb-de74-4782-8dfe-2993ee10560e\"}],\"packageUris\":[\"http://schema.mathworks.com/mf0/Connector/R2020b\"],\"version\":\"1.0\"}"
  Bus Element Out1 : Outport  PortName=Power on

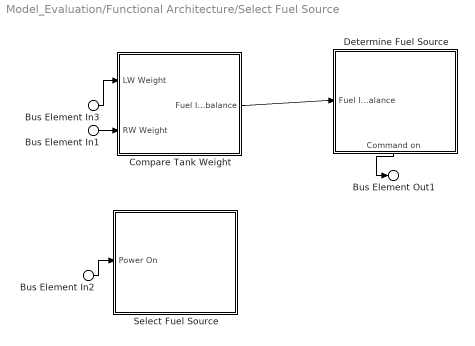
== system Model_Evaluation/Functional Architecture/Select Fuel Source ==
  Bus Element In3 : Inport  PortName=LW Weight
  Bus Element In1 : Inport  Port=2  PortName=RW Weight
  Bus Element In2 : Inport  Port=3  PortName=Power On
  Compare Tank Weight : Subsystem
      settings: PortSchema="{\"entries\":[{\"content\":{\"headerSize\":26,\"margin\":15,\"minimumSpacing\":25,\"sides\":[{\"content\":{\"connectorIds\":[\"In1\",\"In2\"]},\"type\":\"ConnectorPlacement.EquallySpacedRectSide\",\"uuid\":\"40f43dd4-d871-4ec4-b3fe-13d7cd611bac\"},{\"content\":{\"connectorIds\":[\"Out1\"],\"side\":\"RIGHT\"},\"type\":\"ConnectorPlacement.EquallySpacedRectSide\",\"uuid\":\"f931b331-3cfe-490c-8e42-e662817cbd7c\"},{\"content\":{\"connectorIds\":[],\"side\":\"TOP\"},\"type\":\"ConnectorPlacement.EquallySpacedRectSide\",\"uuid\":\"175320fb-a01d-4f5a-a2c2-6f21c6d50255\"}]},\"type\":\"ConnectorPlacement.EquallySpacedConnector\",\"uuid\":\"e178f2bb-de74-4782-8dfe-2993ee10560e\"}],\"packageUris\":[\"http://schema.mathworks.com/mf0/Connector/R2020b\"],\"version\":\"1.0\"}"
  Determine Fuel Source : Subsystem
      settings: PortSchema="{\"entries\":[{\"content\":{\"headerSize\":26,\"margin\":15,\"minimumSpacing\":25,\"sides\":[{\"content\":{\"connectorIds\":[\"In1\"]},\"type\":\"ConnectorPlacement.EquallySpacedRectSide\",\"uuid\":\"40f43dd4-d871-4ec4-b3fe-13d7cd611bac\"},{\"content\":{\"connectorIds\":[],\"side\":\"RIGHT\"},\"type\":\"ConnectorPlacement.EquallySpacedRectSide\",\"uuid\":\"f931b331-3cfe-490c-8e42-e662817cbd7c\"},{\"content\":{\"connectorIds\":[],\"side\":\"TOP\"},\"type\":\"ConnectorPlacement.EquallySpacedRectSide\",\"uuid\":\"175320fb-a01d-4f5a-a2c2-6f21c6d50255\"},{\"content\":{\"connectorIds\":[\"Out1\"],\"side\":\"BOTTOM\"},\"type\":\"ConnectorPlacement.EquallySpacedRectSide\",\"uuid\":\"85e1c832-1027-4f82-8b30-fd110e405833\"}]},\"type\":\"ConnectorPlacement.EquallySpacedConnector\",\"uuid\":\"e178f2bb-de74-4782-8dfe-2993ee10560e\"}],\"packageUris\":[\"http://schema.mathworks.com/mf0/Connector/R2020b\"],\"version\":\"1.0\"}"
  Select Fuel Source : Subsystem
      settings: PortSchema="{\"entries\":[{\"content\":{\"headerSize\":26,\"margin\":15,\"minimumSpacing\":25,\"sides\":[{\"content\":{\"connectorIds\":[\"In1\"]},\"type\":\"ConnectorPlacement.EquallySpacedRectSide\",\"uuid\":\"40f43dd4-d871-4ec4-b3fe-13d7cd611bac\"},{\"content\":{\"connectorIds\":[],\"side\":\"RIGHT\"},\"type\":\"ConnectorPlacement.EquallySpacedRectSide\",\"uuid\":\"f931b331-3cfe-490c-8e42-e662817cbd7c\"},{\"content\":{\"connectorIds\":[],\"side\":\"TOP\"},\"type\":\"ConnectorPlacement.EquallySpacedRectSide\",\"uuid\":\"175320fb-a01d-4f5a-a2c2-6f21c6d50255\"}]},\"type\":\"ConnectorPlacement.EquallySpacedConnector\",\"uuid\":\"e178f2bb-de74-4782-8dfe-2993ee10560e\"}],\"packageUris\":[\"http://schema.mathworks.com/mf0/Connector/R2020b\"],\"version\":\"1.0\"}"
  Bus Element Out1 : Outport  PortName=Command on
  wires:
  Bus Element In3/1 -> Compare Tank Weight/1(LW Weight)
  Bus Element In1/1 -> Compare Tank Weight/2(RW Weight)
  Compare Tank Weight/1(Fuel Imbalance) -> Determine Fuel Source/1(Fuel Imbalance)
  Determine Fuel Source/1(Command on) -> Bus Element Out1/1
  Bus Element In2/1 -> Select Fuel Source/1(Power On)

== system Model_Evaluation/Logical Architecture/Electrical System ==

== system Model_Evaluation/Logical Architecture/Fuel System ==

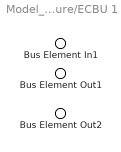
== system Model_Evaluation/Physical Architecture/ECBU 1 ==
  Bus Element In1 : Inport  PortName=InBus
  Bus Element Out1 : Outport  PortName=OutBus
  Bus Element Out2 : Outport  Port=2  PortName=OutBus1

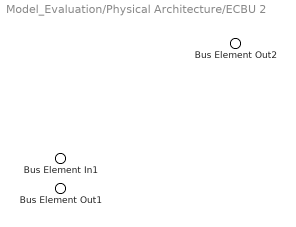
== system Model_Evaluation/Physical Architecture/ECBU 2 ==
  Bus Element In1 : Inport  PortName=InBus
  Bus Element Out2 : Outport  PortName=OutBus1
  Bus Element Out1 : Outport  Port=2  PortName=OutBus

== system Model_Evaluation/Physical Architecture/LH Fuel Qty Sensor 1 ==
  Bus Element Out1 : Outport  PortName=OutBus

== system Model_Evaluation/Physical Architecture/LH Fuel Qty Sensor 2 ==
  Bus Element Out1 : Outport  PortName=OutBus

== system Model_Evaluation/Physical Architecture/LH Fuel Qty Sensor 3 ==
  Bus Element Out1 : Outport  PortName=OutBus

== system Model_Evaluation/Physical Architecture/LH Fuel Qty Sensor 4 ==
  Bus Element Out1 : Outport  PortName=OutBus

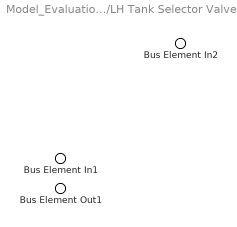
== system Model_Evaluation/Physical Architecture/LH Tank Selector Valve 1 ==
  Bus Element In2 : Inport  PortName=InBus1
  Bus Element In1 : Inport  Port=2  PortName=InBus
  Bus Element Out1 : Outport  PortName=OutBus

== system Model_Evaluation/Physical Architecture/LH Tank Selector Valve 2 ==
  Bus Element In1 : Inport  PortName=InBus
  Bus Element Out1 : Outport  PortName=OutBus

== system Model_Evaluation/Physical Architecture/RH Fuel Qty Sensor 1 ==
  Bus Element Out1 : Outport  PortName=OutBus

== system Model_Evaluation/Physical Architecture/RH Fuel Qty Sensor 2 ==
  Bus Element Out1 : Outport  PortName=OutBus

== system Model_Evaluation/Physical Architecture/RH Fuel Qty Sensor 3 ==
  Bus Element Out1 : Outport  PortName=OutBus

== system Model_Evaluation/Physical Architecture/RH Fuel Qty Sensor 4 ==
  Bus Element Out1 : Outport  PortName=OutBus

== system Model_Evaluation/Physical Architecture/RH Tank Selector Valve 1 ==
  Bus Element In1 : Inport  PortName=InBus
  Bus Element Out1 : Outport  PortName=OutBus

== system Model_Evaluation/Physical Architecture/RH Tank Selector Valve 2 ==
  Bus Element In1 : Inport  PortName=InBus
  Bus Element Out1 : Outport  PortName=OutBus

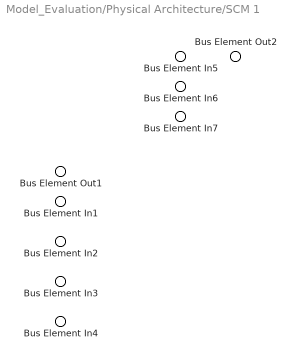
== system Model_Evaluation/Physical Architecture/SCM 1 ==
  Bus Element In6 : Inport  PortName=InBus5
  Bus Element In7 : Inport  Port=2  PortName=InBus6
  Bus Element In5 : Inport  Port=3  PortName=InBus4
  Bus Element In1 : Inport  Port=4  PortName=InBus
  Bus Element In2 : Inport  Port=5  PortName=InBus1
  Bus Element In3 : Inport  Port=6  PortName=InBus2
  Bus Element In4 : Inport  Port=7  PortName=InBus3
  Bus Element Out2 : Outport  PortName=OutBus1
  Bus Element Out1 : Outport  Port=2  PortName=OutBus

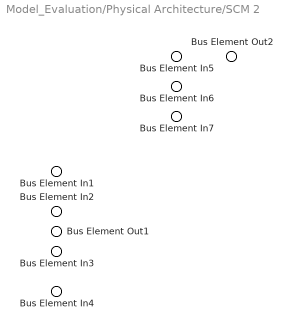
== system Model_Evaluation/Physical Architecture/SCM 2 ==
  Bus Element In7 : Inport  PortName=InBus6
  Bus Element In6 : Inport  Port=2  PortName=InBus5
  Bus Element In5 : Inport  Port=3  PortName=InBus4
  Bus Element In1 : Inport  Port=4  PortName=InBus
  Bus Element In2 : Inport  Port=5  PortName=InBus1
  Bus Element In3 : Inport  Port=6  PortName=InBus2
  Bus Element In4 : Inport  Port=7  PortName=InBus3
  Bus Element Out2 : Outport  PortName=OutBus1
  Bus Element Out1 : Outport  Port=2  PortName=OutBus

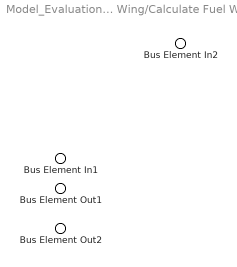
== system Model_Evaluation/Functional Architecture/ Determine Fuel Weight per Wing/Calculate Fuel Weight ==
  Bus Element In2 : Inport  PortName=LH Level
  Bus Element In1 : Inport  Port=2  PortName=RH Level
  Bus Element Out1 : Outport  PortName=LW Weight
  Bus Element Out2 : Outport  Port=2  PortName=RW Weight

== system Model_Evaluation/Functional Architecture/ Determine Fuel Weight per Wing/Sense LH Wing Fuel Level ==
  Bus Element Out1 : Outport  PortName=LH Level

== system Model_Evaluation/Functional Architecture/ Determine Fuel Weight per Wing/Sense RH Wing Fuel Level ==
  Bus Element Out1 : Outport  PortName=RH Level

== system Model_Evaluation/Functional Architecture/Provide Electrical Power/Control Power to Loads ==

== system Model_Evaluation/Functional Architecture/Provide Electrical Power/Protect Bus from High Current Condtion ==

== system Model_Evaluation/Functional Architecture/Provide Electrical Power/Protect Bus from High Voltage Condition ==

== system Model_Evaluation/Functional Architecture/Select Fuel Source/Compare Tank Weight ==
  Bus Element In1 : Inport  PortName=LW Weight
  Bus Element In2 : Inport  Port=2  PortName=RW Weight
  Bus Element Out1 : Outport  PortName=Fuel Imbalance

== system Model_Evaluation/Functional Architecture/Select Fuel Source/Determine Fuel Source ==
  Bus Element In1 : Inport  PortName=Fuel Imbalance
  Bus Element Out1 : Outport  PortName=Command on

== system Model_Evaluation/Functional Architecture/Select Fuel Source/Select Fuel Source ==
  Bus Element In1 : Inport  PortName=Power On
